simulink model "PID_simulink"  (R2022b)
settings: Solver=VariableStepAuto  StartTime=0.0  StopTime=30  RelTol=1e-3
libraries: simulink x1
settings Model: Creator=USER  LastModifiedBy=USER

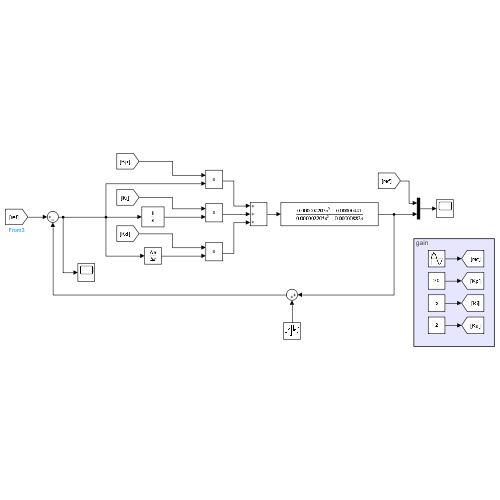
[thumbnail: Simulink's stored preview of the top-level diagram]
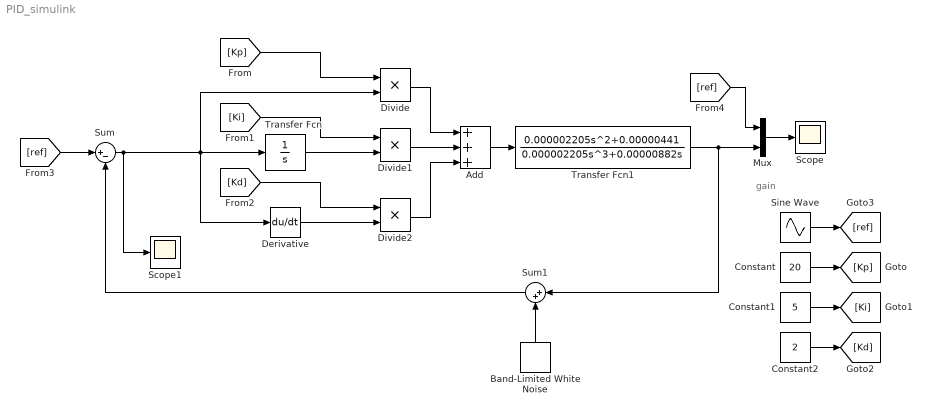
== system PID_simulink ==
  note: gain
  Add : Sum  Inputs=+++
  Band-Limited White Noise : simulink/Sources/Band-Limited White Noise  Cov=[0.1]  Ts=0.1  seed=[23341]
  Constant : Constant  Value=20
  Constant1 : Constant  Value=5
  Constant2 : Constant  Value=2
  Derivative : Derivative
  Divide : Product  Inputs=**
  Divide1 : Product  Inputs=**
  Divide2 : Product  Inputs=**
  Mux : Mux  Inputs=2
  Scope : Scope
  Scope1 : Scope
  Sine Wave : Sin  Amplitude=10  Frequency=0.4  SampleTime=0
  Sum : Sum  Inputs=|+-
  Sum1 : Sum  Inputs=|++
  Transfer Fcn : TransferFcn  Denominator=[1 0]
  Transfer Fcn1 : TransferFcn  Numerator=[0.000002205 0 0.00000441]  Denominator=[0.000002205 0 0.00000882 0]
  wires:
  Sum/1 -> Scope1/1, Derivative/1, Transfer Fcn/1, Divide/2
  Constant/1 -> [Kp]
  Constant1/1 -> [Ki]
  Constant2/1 -> [Kd]
  [Kp] -> Divide/1
  [Ki] -> Divide1/1
  [Kd] -> Divide2/1
  Transfer Fcn/1 -> Divide1/2
  Derivative/1 -> Divide2/2
  Sine Wave/1 -> [ref]
  Divide1/1 -> Add/2
  Divide/1 -> Add/1
  Divide2/1 -> Add/3
  Mux/1 -> Scope/1
  Add/1 -> Transfer Fcn1/1
  [ref] -> Mux/1
  Transfer Fcn1/1 -> Sum1/1, Mux/2
  [ref] -> Sum/1
  Sum1/1 -> Sum/2
  Band-Limited White Noise/1 -> Sum1/2
